simulink model "hexacopter"  (R2019a)
settings: Solver=ode4  StartTime=0.0  StopTime=10.0  FixedStep=0.01  RelTol=1e-3  EnableMultiTasking=on
settings Model: Creator=fmina  LastModifiedBy=Yifei
settings DataIOCC: ReturnWorkspaceOutputs=off
settings OptimizationCC: LifeSpan=inf
settings DebuggingCC: SFUnexpectedBacktrackingDiag=warning  SFNoUnconditionalDefaultTransitionDiag=warning  SFExecutionAtInitializationDiag=none  ArithmeticOperatorsInVariantConditions=warning
settings SFSimCC: SimUseLocalCustomCode=off
settings RTWCC: RTWUseLocalCustomCode=off
settings CodeAppCC: StateflowObjectComments=on
settings GRTTargetCC: TargetLangStandard=C89/C90 (ANSI)  GeneratePreprocessorConditionals=Disable all
settings ConfigComp: CovMetricSettings=dw  CovHtmlReporting=on  CovSaveCumulativeToWorkspaceVar=on  CovSaveSingleToWorkspaceVar=on  CovExternalEMLEnable=off

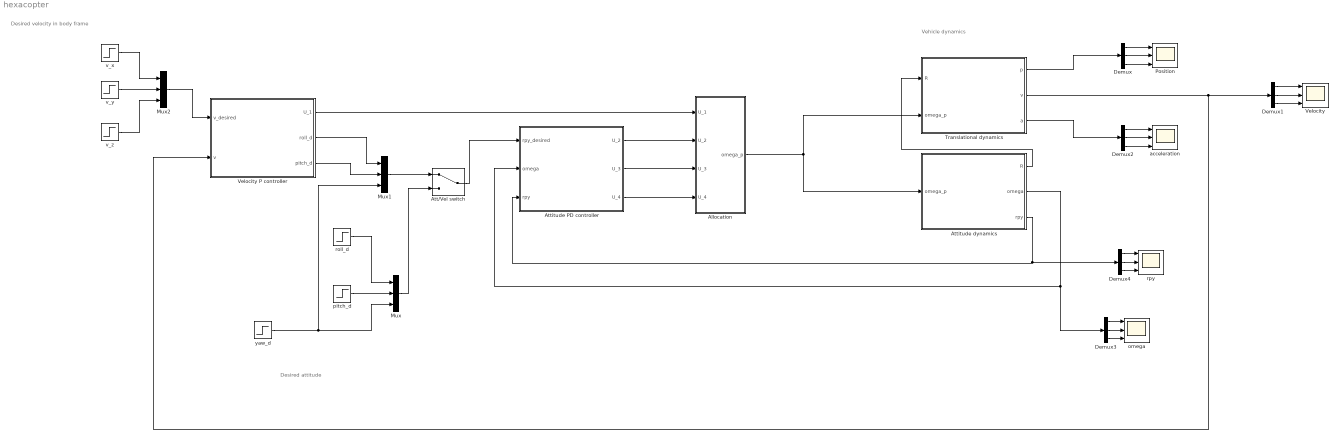
== system hexacopter ==
  note: Desired velocity in body frame
  note: Vehicle dynamics
  note: Desired attitude
  Allocation : Subsystem
  Att/Vel switch : ManualSwitch
  Attitude PD controller : Subsystem
  Attitude dynamics : Subsystem
  Demux{,1..4} (5 alike) : Demux  Outputs=3
  Mux : Mux  Inputs=3
  Mux1 : Mux  Inputs=3
  Mux2 : Mux  Inputs=3
  Position : Scope  NumInputPorts=3
  Translational dynamics : Subsystem
  Velocity : Scope  NumInputPorts=3
  Velocity P controller : Subsystem
  acceleration : Scope  NumInputPorts=3
  omega : Scope  NumInputPorts=3
  pitch_d : Step  Time=3  After=0.25  SampleTime=0
  roll_d : Step  After=0.24  SampleTime=0
  rpy : Scope  NumInputPorts=3
  v_x : Step  SampleTime=0
  v_y : Step  Time=3  After=0.4  SampleTime=0
  v_z : Step  Time=5  After=0  SampleTime=0
  yaw_d : Step  Time=5  After=0  SampleTime=0
  wires:
  Demux/2 -> Position/2
  Demux/3 -> Position/3
  Demux/1 -> Position/1
  Demux1/2 -> Velocity/2
  Demux1/3 -> Velocity/3
  Demux1/1 -> Velocity/1
  Demux2/2 -> acceleration/2
  Demux2/3 -> acceleration/3
  Demux2/1 -> acceleration/1
  Demux3/2 -> omega/2
  Demux3/3 -> omega/3
  Demux3/1 -> omega/1
  Demux4/1 -> rpy/1
  Demux4/2 -> rpy/2
  Demux4/3 -> rpy/3
  roll_d/1 -> Mux/1
  pitch_d/1 -> Mux/2
  yaw_d/1 -> Mux/3, Mux1/3
  Att/Vel switch/1 -> Attitude PD controller/1(rpy_desired)
  Velocity P controller/3(pitch_d) -> Mux1/2
  Velocity P controller/2(roll_d) -> Mux1/1
  Mux/1 -> Att/Vel switch/2
  Mux1/1 -> Att/Vel switch/1
  Mux2/1 -> Velocity P controller/1(v_desired)
  v_x/1 -> Mux2/1
  v_y/1 -> Mux2/2
  v_z/1 -> Mux2/3
  Allocation/1(omega_p) -> Attitude dynamics/1(omega_p), Translational dynamics/2(omega_p)
  Velocity P controller/1(U_1) -> Allocation/1(U_1)
  Attitude PD controller/1(U_2) -> Allocation/2(U_2)
  Attitude PD controller/2(U_3) -> Allocation/3(U_3)
  Attitude PD controller/3(U_4) -> Allocation/4(U_4)
  Attitude dynamics/1(R) -> Translational dynamics/1(R)
  Attitude dynamics/2(omega) -> Demux3/1, Attitude PD controller/2("omega ")
  Attitude dynamics/3(rpy) -> Attitude PD controller/3(rpy), Demux4/1
  Translational dynamics/3(a) -> Demux2/1
  Translational dynamics/1(p) -> Demux/1
  Translational dynamics/2(v) -> Velocity P controller/2(v), Demux1/1

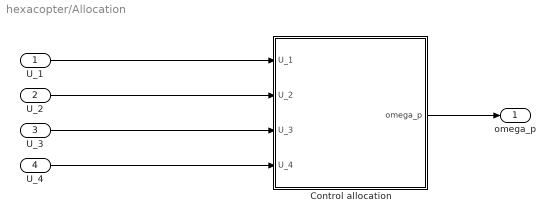
== system hexacopter/Allocation ==
  U_1 : Inport
  U_2 : Inport  Port=2
  U_3 : Inport  Port=3
  U_4 : Inport  Port=4
  Control allocation : MATLAB Function  TreatAsAtomicUnit=on
  omega_p : Outport  PortDimensions=[6,1]
  wires:
  U_1/1 -> Control allocation/1(U_1)
  Control allocation/1(omega_p) -> omega_p/1
  U_4/1 -> Control allocation/4(U_4)
  U_2/1 -> Control allocation/2(U_2)
  U_3/1 -> Control allocation/3(U_3)

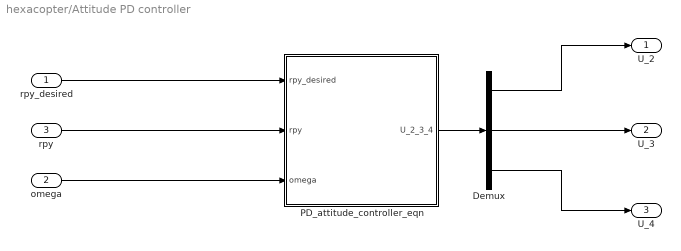
== system hexacopter/Attitude PD controller ==
  rpy_desired : Inport
  "omega " : Inport  Port=2
  rpy : Inport  Port=3
  Demux : Demux  Outputs=3
  PD_attitude_controller_eqn : MATLAB Function  TreatAsAtomicUnit=on
  U_2 : Outport
  U_3 : Outport  Port=2
  U_4 : Outport  Port=3
  wires:
  rpy_desired/1 -> PD_attitude_controller_eqn/1(rpy_desired)
  rpy/1 -> PD_attitude_controller_eqn/2(rpy)
  "omega "/1 -> PD_attitude_controller_eqn/3(omega)
  PD_attitude_controller_eqn/1(U_2_3_4) -> Demux/1
  Demux/1 -> U_2/1
  Demux/2 -> U_3/1
  Demux/3 -> U_4/1

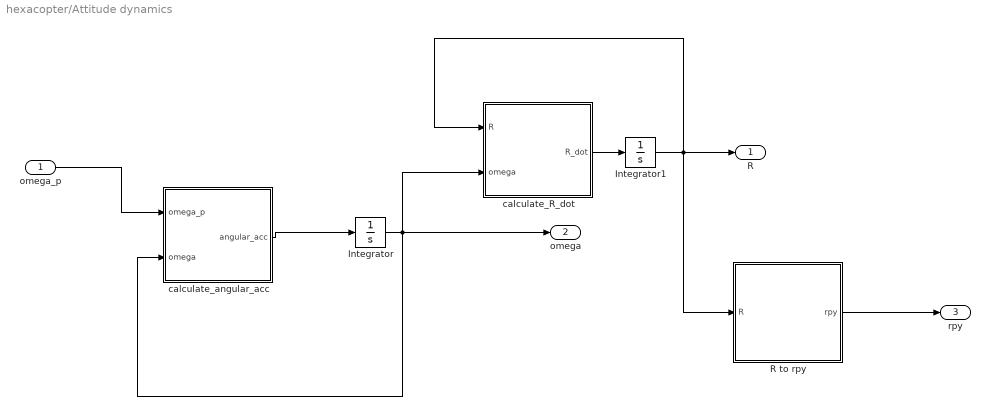
== system hexacopter/Attitude dynamics ==
  omega_p : Inport
  Integrator : Integrator  InitialCondition=zeros(3,1)
  Integrator1 : Integrator  InitialCondition=eye(3)
  R to rpy : MATLAB Function  TreatAsAtomicUnit=on
  calculate_R_dot : MATLAB Function  TreatAsAtomicUnit=on
  calculate_angular_acc : MATLAB Function  TreatAsAtomicUnit=on
  R : Outport
  omega : Outport  Port=2
  rpy : Outport  Port=3
  wires:
  omega_p/1 -> calculate_angular_acc/1(omega_p)
  calculate_angular_acc/1(angular_acc) -> Integrator/1
  Integrator/1 -> calculate_R_dot/2(omega), calculate_angular_acc/2(omega), omega/1
  calculate_R_dot/1(R_dot) -> Integrator1/1
  R to rpy/1(rpy) -> rpy/1
  Integrator1/1 -> R to rpy/1(R), calculate_R_dot/1(R), R/1

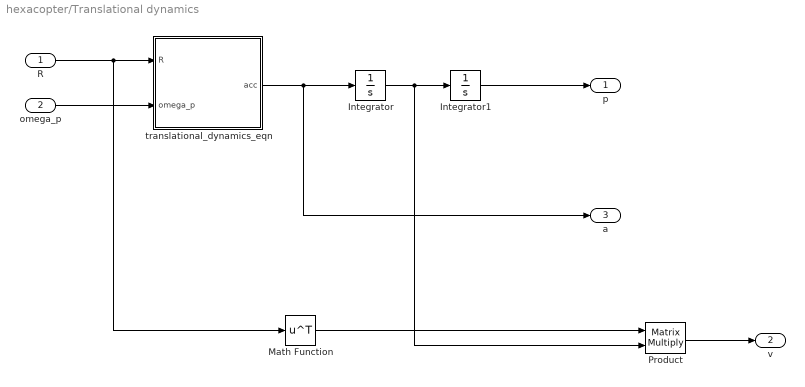
== system hexacopter/Translational dynamics ==
  R : Inport
  omega_p : Inport  Port=2
  Integrator : Integrator
  Integrator1 : Integrator
  Math Function : Math  Operator=transpose  SaturateOnIntegerOverflow=on
  Product : Product  Multiplication=Matrix(*)
  translational_dynamics_eqn : MATLAB Function  TreatAsAtomicUnit=on
  p : Outport
  v : Outport  Port=2
  a : Outport  Port=3
  wires:
  translational_dynamics_eqn/1(acc) -> a/1, Integrator/1
  Integrator/1 -> Product/2, Integrator1/1
  Integrator1/1 -> p/1
  omega_p/1 -> translational_dynamics_eqn/2(omega_p)
  R/1 -> Math Function/1, translational_dynamics_eqn/1(R)
  Math Function/1 -> Product/1
  Product/1 -> v/1

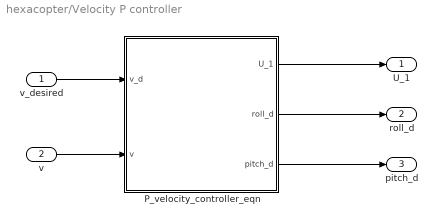
== system hexacopter/Velocity P controller ==
  v_desired : Inport
  v : Inport  Port=2
  P_velocity_controller_eqn : MATLAB Function  TreatAsAtomicUnit=on
  U_1 : Outport
  roll_d : Outport  Port=2
  pitch_d : Outport  Port=3
  wires:
  v_desired/1 -> P_velocity_controller_eqn/1(v_d)
  v/1 -> P_velocity_controller_eqn/2(v)
  P_velocity_controller_eqn/1(U_1) -> U_1/1
  P_velocity_controller_eqn/3(pitch_d) -> pitch_d/1
  P_velocity_controller_eqn/2(roll_d) -> roll_d/1

== matlab function hexacopter/Attitude dynamics/calculate_angular_acc ==
  data: omega_p input; angular_acc output; omega input
function angular_acc = fcn(omega_p, omega)
%omega_p is the rotational speed of the propellers. This vector must have
%size 6.
%omega is the angular velocity of the MAV expressed in body frame.

%load parameters
%Inertia is found under params.J
params = parameters();


U = params.allocation_matrix*(omega_p.^2);
angular_acc = inv(params.J)*(-cross(omega, params.J*omega) + U(2:4));

== matlab function hexacopter/Translational dynamics/translational_dynamics_eqn ==
  data: R input; acc output; omega_p input
function acc = fcn(R, omega_p)

%load parameters
% to access for instance vehicle mass, use params.m.
% accelerational gravity is under params.g
params = parameters();

U = params.allocation_matrix*(omega_p.^2);

%acceleration is given by:
acc = params.g + [0;0;U(1)/params.m];

end

== matlab function hexacopter/Attitude dynamics/calculate_R_dot ==
  data: R input; R_dot output; omega input
function R_dot = fcn(R, omega)

%load parameters
params = parameters();

%normalize R every step to guarantee that R is orthogonal matrix (valid
%rotation)
[U,~,V] = svd(R);
R = U*V';

%Write R_dot = R*skew_omega
R_dot = R*[0 -omega(3) omega(2); omega(3) 0 -omega(1); -omega(2) omega(1) 0];

== matlab function hexacopter/Attitude dynamics/R to rpy ==
  data: R input; rpy output
function rpy = fcn(R)

%calculate roll pitch yaw from rotation matrix

pitch = asin(-R(3,1));
roll = atan2(R(3,2), R(3,3));
yaw = atan2(R(2,1), R(1,1));

rpy = [roll; pitch; yaw];

== matlab function hexacopter/Attitude PD controller/PD_attitude_controller_eqn ==
  data: rpy_desired input; U_2_3_4 output; rpy input; omega input
function U_2_3_4 = fcn(rpy_desired, rpy, omega)

%load parameters
%controller Kp is found under params.attitude_Kp
%controller Kd is found under params.attitude_Kd
params = parameters();
Kp = params.attitude_Kp;
Kd = params.attitude_Kd;
roll = rpy(1);
pitch = rpy(2);
yaw = rpy(3);

%control error is given by
% error = ...; (Complete here)

% Relation between Tait-Bryan angles and angular velocities
%E_r = ...; (Complete here)


% rpy_dot = ...; (from omega in body frame)


%control action U_2_3_4 = [U_2, U_3, U_4] is given by
U_2_3_4 = (rpy_desired - rpy).*Kp - omega.*Kd;

== matlab function hexacopter/Velocity P controller/P_velocity_controller_eqn ==
  data: v_d input; U_1 output; v input; roll_d output; pitch_d output
function [U_1, roll_d, pitch_d] = fcn(v_d, v)

%load parameters
%controller Kp is found under params.velocity_Kp
params = parameters();
Kp = params.velocity_Kp;
%control error is given by 
error = v_d - v;

%control action is given by
U_1 = 0;
roll_d = 0;
pitch_d = 0;

U_1 = error*Kp/; 
%roll_d = ...;
%pitch_d = ...;

== matlab function hexacopter/Allocation/Control allocation ==
  data: U_1 input; omega_p output; U_2 input; U_3 input; U_4 input
function omega_p = fcn(U_1, U_2, U_3, U_4)

%load parameters
params = parameters();

omega_p_sqr = params.pinv_allocation_matrix*[U_1; U_2; U_3; U_4];

%make sure only positive values are allowed.
omega_p_sqr = max(omega_p_sqr, zeros(6,1));

%actual rotors velocities
omega_p = sqrt(omega_p_sqr);
